simulink model "Inverter_with_mean_losses"  (R2022b)
settings: configuration reference "ModelConfig_var" (kept outside this file)
InitFcn:
  | %% BUS initialization
  | Xabc.A = 0;
  | Xabc.B = 0;
  | Xabc.C = 0;
  | % -------------------------------------------------------------------------
  | Simulink.Bus.createObject(Xabc)
  | XabcBus = slBus1;
  | clear slBus1
undefined symbols (not defined in the file): InputCircuit, InverterParams, TimeSteps
settings Model: Creator=KIRTACA  LastModifiedBy=FAGNAL
settings ConfigSetRef: SourceName=ModelConfig_var  SourceLocation=Base Workspace

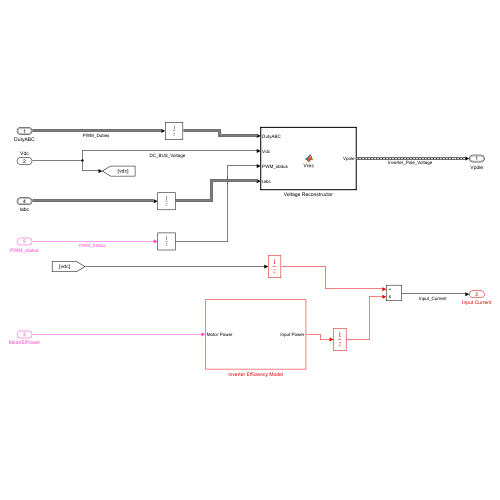
[thumbnail: Simulink's stored preview of the top-level diagram]
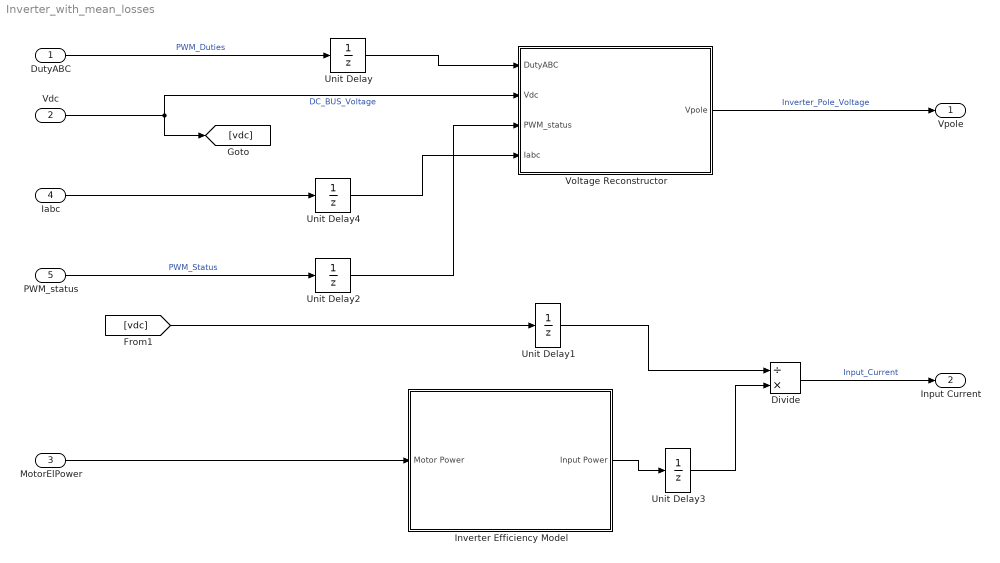
== system Inverter_with_mean_losses ==
  DutyABC : Inport  OutDataTypeStr=Bus: XabcBus
  Vdc : Inport  Port=2
  MotorElPower : Inport  Port=3
  Iabc : Inport  Port=4  OutDataTypeStr=Bus: XabcBus
  PWM_status : Inport  Port=5
  Divide : Product  Inputs=/*
  Inverter Efficiency Model : Subsystem
  Unit Delay{,2..4} (4 alike) : UnitDelay  SampleTime=-1  HasFrameUpgradeWarning=on
  Unit Delay1 : UnitDelay  InitialCondition=InputCircuit.Vdc_i  SampleTime=-1  HasFrameUpgradeWarning=on
  Voltage Reconstructor : MATLAB Function  TreatAsAtomicUnit=on  mask{Vce=InverterParams.Vce, Vfd=InverterParams.Vfd, RonT=InverterParams.RonT, RonD=InverterParams.RonD, Rshunt=InverterParams.Rshunt, tdt=InverterParams.tdt, tau=InverterParams.tau, tsw=TimeSteps.ModelStep}
      mask prompts: Vce "Vce IGBT[V]"; Vfd "Vfd Diode [V]"; RonT "RonT IGBT [Ohm]"; RonD "RonD  Diode[Ohm]"; Rshunt "Rshunt [Ohm]"; tdt "Deadtime [s]"; tau "Tau [s]"; tsw "Pwm Time [s]"
  "Vpole " : Outport  OutDataTypeStr=Bus: XabcBus  VectorParamsAs1DForOutWhenUnconnected=off
  Input Current : Outport  Port=2  VectorParamsAs1DForOutWhenUnconnected=off
  wires:
  Inverter Efficiency Model/1(Input Power) -> Unit Delay3/1
  Unit Delay3/1 -> Divide/2
  Unit Delay1/1 -> Divide/1
  [vdc] -> Unit Delay1/1
  DutyABC/1 -> Unit Delay/1  "PWM_Duties"
  Vdc/1 -> Voltage Reconstructor/2(Vdc), [vdc]  "DC_BUS_Voltage"
  MotorElPower/1 -> Inverter Efficiency Model/1(Motor Power)
  Divide/1 -> Input Current/1  "Input_Current"
  Voltage Reconstructor/1(Vpole) -> "Vpole "/1  "Inverter_Pole_Voltage"
  Iabc/1 -> Unit Delay4/1
  PWM_status/1 -> Unit Delay2/1  "PWM_Status"
  Unit Delay/1 -> Voltage Reconstructor/1(DutyABC)
  Unit Delay2/1 -> Voltage Reconstructor/3(PWM_status)
  Unit Delay4/1 -> Voltage Reconstructor/4(Iabc)

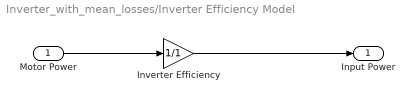
== system Inverter_with_mean_losses/Inverter Efficiency Model ==
  Motor Power : Inport
  Inverter Efficiency : Gain  Gain=1/1
  Input Power : Outport  VectorParamsAs1DForOutWhenUnconnected=off
  wires:
  Motor Power/1 -> Inverter Efficiency/1
  Inverter Efficiency/1 -> Input Power/1

== matlab function Inverter_with_mean_losses/Voltage Reconstructor ==
  data: DutyABC input Bus: XabcBus size=1; Vpole output Bus: XabcBus size=1; Vdc input; PWM_status input; Iabc input; Vce parameter; Vfd parameter; RonT parameter; Rshunt parameter; tdt parameter; tau parameter; tsw parameter; RonD parameter
function Vpole   = Vrec(DutyABC, Vdc, PWM_status, Iabc, Vce, Vfd, RonT, Rshunt, tdt, tau, tsw, RonD)

sigm = @(x) (1-exp(-x/tau));

if (PWM_status == 1)
    
    Da = DutyABC.A;
    Db = DutyABC.B;
    Dc = DutyABC.C;
    
    Vpole_v = zeros(1,3);
    Iin = zeros(1,3);
    DutyABC_v = zeros(1,3);
    
    Iin(1) = Iabc.A;
    Iin(2) = Iabc.B;
    Iin(3) = Iabc.C;
    
    DutyABC_v(1) = Da;
    DutyABC_v(2) = Db;
    DutyABC_v(3) = Dc;

    for i=1:3

        I = abs(Iin(i));

        if Iin(i)>=0
            D = DutyABC_v(i) - tdt/tsw * sigm(I);
            Vpole_v(i) = D *Vdc - D*(Vce+RonT*I)-(1-D)*(Vfd+(RonD+Rshunt)*I);
        else
            D = DutyABC_v(i) + tdt/tsw * sigm(I);
            Vpole_v(i) = D *Vdc+ D*(Vfd+RonD*I)+(1-D)*(Vce+(RonT+Rshunt)*I);

        end
    end    
    Vpole.A = Vpole_v(1);
    Vpole.B = Vpole_v(2);
    Vpole.C = Vpole_v(3);
else
    Da = 0.5;
    Db = 0.5;
    Dc = 0.5;

    Vpole.A = Vdc * Da;
    Vpole.B = Vdc * Db;
    Vpole.C = Vdc * Dc;
end
